simulink model "TST_FlFWLvl_DD"  (R2016b)
settings: Solver=FixedStepDiscrete  StartTime=0.0  StopTime=simTime  FixedStep=sampleTime  RelTol=1e-3
values from neighbouring files (symbols this model uses):
  testCase = 1    [initTST_FlFWLvl_DD_001.m]
libraries: simulink x4, UnitTest_Lib x2
settings Model: Creator=liutao  LastModifiedBy=liutao
settings DebuggingCC: SignalRangeChecking=error

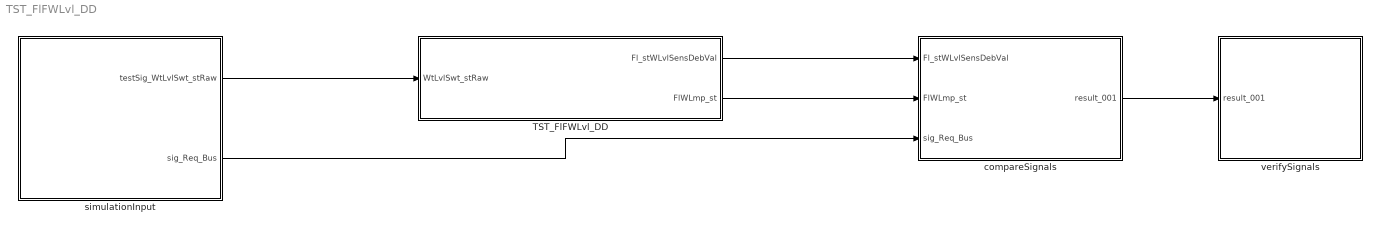
== system TST_FlFWLvl_DD ==
  TST_FlFWLvl_DD : Subsystem
  compareSignals : Subsystem
  simulationInput : Subsystem
  verifySignals : Subsystem
  wires:
  simulationInput/1(testSig_WtLvlSwt_stRaw) -> TST_FlFWLvl_DD/1(WtLvlSwt_stRaw)
  TST_FlFWLvl_DD/1(Fl_stWLvlSensDebVal) -> compareSignals/1(Fl_stWLvlSensDebVal)
  TST_FlFWLvl_DD/2(FlWLmp_st) -> compareSignals/2(FlWLmp_st)
  simulationInput/2(sig_Req_Bus) -> compareSignals/3(sig_Req_Bus)
  compareSignals/1(result_001) -> verifySignals/1(result_001)

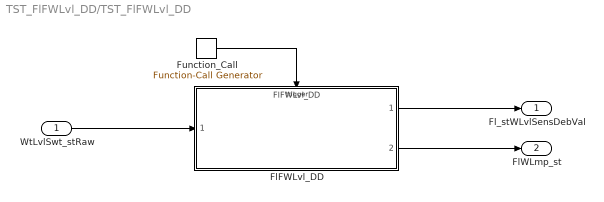
== system TST_FlFWLvl_DD/TST_FlFWLvl_DD ==
  WtLvlSwt_stRaw : Inport
  FlFWLvl_DD : ModelReference  ModelNameDialog=FlFWLvl_DD  SimulationMode=Normal  ModelReferenceVersion=1.14  TriggerPortName=function  TriggerPortTriggerType=function-call  TriggerPortStatesWhenEnabling=held
  Function_Call : simulink/Ports & Subsystems/Function-Call Generator  sample_time=sampleTime  numberOfIterations=1
  Fl_stWLvlSensDebVal : Outport
  FlWLmp_st : Outport  Port=2
  wires:
  Function_Call/1 -> FlFWLvl_DD/Trigger
  WtLvlSwt_stRaw/1 -> FlFWLvl_DD/1
  FlFWLvl_DD/1 -> Fl_stWLvlSensDebVal/1
  FlFWLvl_DD/2 -> FlWLmp_st/1

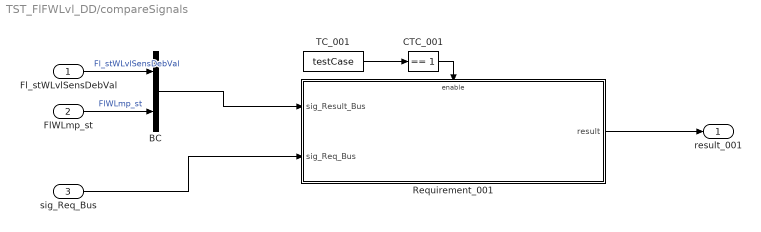
== system TST_FlFWLvl_DD/compareSignals ==
  Fl_stWLvlSensDebVal : Inport
  FlWLmp_st : Inport  Port=2
  sig_Req_Bus : Inport  Port=3
  BC : BusCreator  Inputs=2
  CTC_001 : simulink/Logic and Bit Operations/Compare To Constant  relop===  const=1  OutDataTypeStr=boolean
  Requirement_001 : Subsystem
  TC_001 : Constant  Value=testCase
  result_001 : Outport
  wires:
  Fl_stWLvlSensDebVal/1 -> BC/1  "Fl_stWLvlSensDebVal"
  FlWLmp_st/1 -> BC/2  "FlWLmp_st"
  TC_001/1 -> CTC_001/1
  CTC_001/1 -> Requirement_001/Enable
  sig_Req_Bus/1 -> Requirement_001/2(sig_Req_Bus)
  BC/1 -> Requirement_001/1(sig_Result_Bus)
  Requirement_001/1(result) -> result_001/1

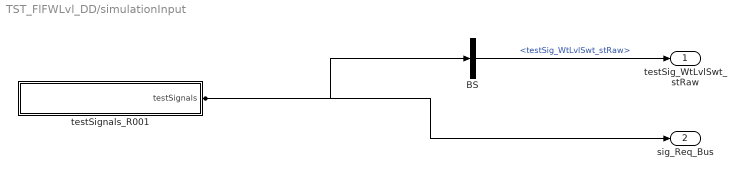
== system TST_FlFWLvl_DD/simulationInput ==
  BS : BusSelector  OutputSignals=testSig_WtLvlSwt_stRaw
  testSignals_R001 : Subsystem
  testSig_WtLvlSwt_stRaw : Outport
  sig_Req_Bus : Outport  Port=2
  wires:
  BS/1 -> testSig_WtLvlSwt_stRaw/1  "<testSig_WtLvlSwt_stRaw>"
  testSignals_R001/1(testSignals) -> BS/1, sig_Req_Bus/1

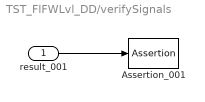
== system TST_FlFWLvl_DD/verifySignals ==
  result_001 : Inport
  Assertion_001 : Assertion  Enabled=off
  wires:
  result_001/1 -> Assertion_001/1

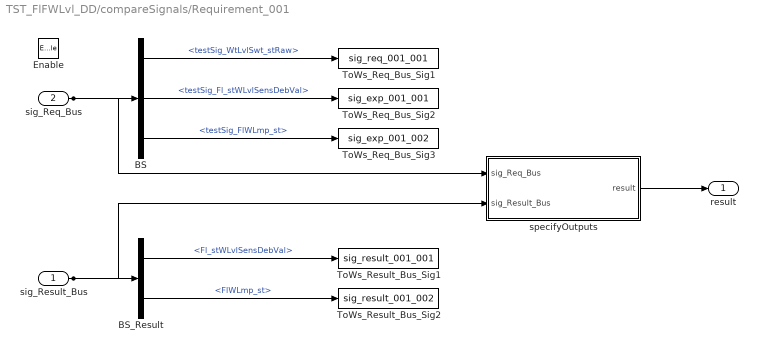
== system TST_FlFWLvl_DD/compareSignals/Requirement_001 ==
  sig_Result_Bus : Inport
  sig_Req_Bus : Inport  Port=2
  Enable : EnablePort
  BS : BusSelector  OutputSignals=testSig_WtLvlSwt_stRaw,testSig_Fl_stWLvlSensDebVal,testSig_FlWLmp_st
  BS_Result : BusSelector  OutputSignals=Fl_stWLvlSensDebVal,FlWLmp_st
  ToWs_Req_Bus_Sig1 : ToWorkspace  VariableName=sig_req_001_001  SaveFormat=Structure With Time
  ToWs_Req_Bus_Sig2 : ToWorkspace  VariableName=sig_exp_001_001  SaveFormat=Structure With Time
  ToWs_Req_Bus_Sig3 : ToWorkspace  VariableName=sig_exp_001_002  SaveFormat=Structure With Time
  ToWs_Result_Bus_Sig1 : ToWorkspace  VariableName=sig_result_001_001  SaveFormat=Structure With Time
  ToWs_Result_Bus_Sig2 : ToWorkspace  VariableName=sig_result_001_002  SaveFormat=Structure With Time
  specifyOutputs : Subsystem
  result : Outport
  wires:
  sig_Req_Bus/1 -> BS/1, specifyOutputs/1(sig_Req_Bus)
  BS/1 -> ToWs_Req_Bus_Sig1/1  "<testSig_WtLvlSwt_stRaw>"
  BS/2 -> ToWs_Req_Bus_Sig2/1  "<testSig_Fl_stWLvlSensDebVal>"
  BS/3 -> ToWs_Req_Bus_Sig3/1  "<testSig_FlWLmp_st>"
  sig_Result_Bus/1 -> BS_Result/1, specifyOutputs/2(sig_Result_Bus)
  BS_Result/1 -> ToWs_Result_Bus_Sig1/1  "<Fl_stWLvlSensDebVal>"
  BS_Result/2 -> ToWs_Result_Bus_Sig2/1  "<FlWLmp_st>"
  specifyOutputs/1(result) -> result/1

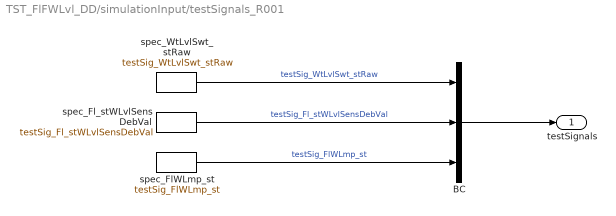
== system TST_FlFWLvl_DD/simulationInput/testSignals_R001 ==
  BC : BusCreator  Inputs=3
  spec_FlWLmp_st : FromWorkspace  VariableName=testSig_FlWLmp_st  Interpolate=off  OutputAfterFinalValue=Holding final value
  spec_Fl_stWLvlSensDebVal : FromWorkspace  VariableName=testSig_Fl_stWLvlSensDebVal  Interpolate=off  OutputAfterFinalValue=Holding final value
  spec_WtLvlSwt_stRaw : FromWorkspace  VariableName=testSig_WtLvlSwt_stRaw  Interpolate=off  OutputAfterFinalValue=Holding final value
  testSignals : Outport
  wires:
  BC/1 -> testSignals/1
  spec_WtLvlSwt_stRaw/1 -> BC/1  "testSig_WtLvlSwt_stRaw"
  spec_Fl_stWLvlSensDebVal/1 -> BC/2  "testSig_Fl_stWLvlSensDebVal"
  spec_FlWLmp_st/1 -> BC/3  "testSig_FlWLmp_st"

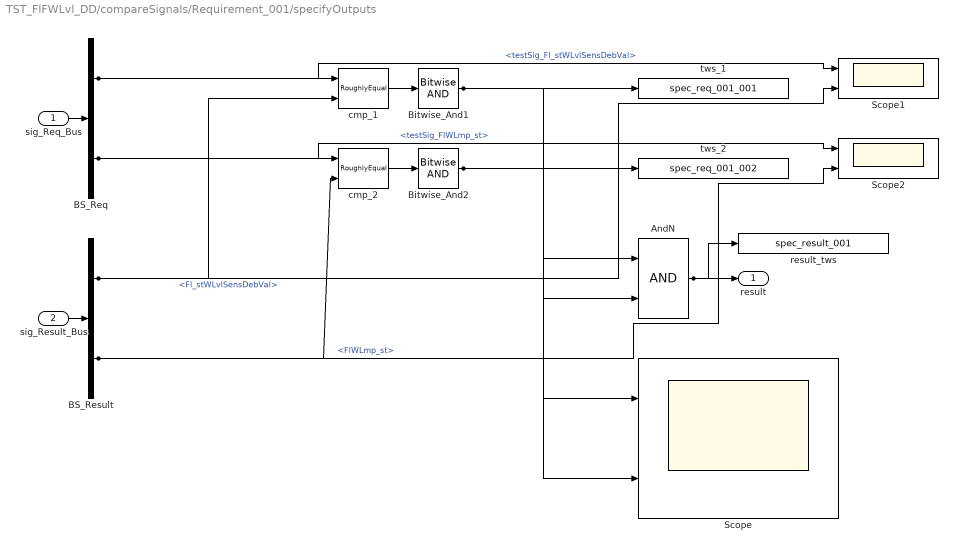
== system TST_FlFWLvl_DD/compareSignals/Requirement_001/specifyOutputs ==
  sig_Req_Bus : Inport
  sig_Result_Bus : Inport  Port=2
  AndN : Logic
  BS_Req : BusSelector  OutputSignals=testSig_Fl_stWLvlSensDebVal,testSig_FlWLmp_st
  BS_Result : BusSelector  OutputSignals=Fl_stWLvlSensDebVal,FlWLmp_st
  Bitwise_And1 : simulink/Logic and Bit Operations/Bitwise Operator  logicop=AND  UseBitMask=off  BitMask=bin2dec('11011001')  BitMaskRealWorld=Stored Integer
  Bitwise_And2 : simulink/Logic and Bit Operations/Bitwise Operator  logicop=AND  UseBitMask=off  BitMask=bin2dec('11011001')  BitMaskRealWorld=Stored Integer
  Scope : Scope  NumInputPorts=2
  Scope1 : Scope  NumInputPorts=2
  Scope2 : Scope  NumInputPorts=2
  cmp_1 : UnitTest_Lib/RoughlyEqual  slope=0.1
  cmp_2 : UnitTest_Lib/RoughlyEqual  slope=0.1
  result_tws : ToWorkspace  VariableName=spec_result_001
  tws_1 : ToWorkspace  VariableName=spec_req_001_001
  tws_2 : ToWorkspace  VariableName=spec_req_001_002
  result : Outport
  wires:
  sig_Req_Bus/1 -> BS_Req/1
  sig_Result_Bus/1 -> BS_Result/1
  AndN/1 -> result/1, result_tws/1
  BS_Req/1 -> cmp_1/1, Scope1/1  "<testSig_Fl_stWLvlSensDebVal>"
  BS_Result/1 -> cmp_1/2, Scope1/2  "<Fl_stWLvlSensDebVal>"
  cmp_1/1 -> Bitwise_And1/1
  Bitwise_And1/1 -> tws_1/1, AndN/1, Scope/1
  BS_Req/2 -> cmp_2/1, Scope2/1  "<testSig_FlWLmp_st>"
  BS_Result/2 -> cmp_2/2, Scope2/2  "<FlWLmp_st>"
  cmp_2/1 -> Bitwise_And2/1
  Bitwise_And2/1 -> tws_2/1, AndN/2, Scope/2
